simulink model "digitalControlSim"  (R2020a)
settings: Solver=VariableStepAuto  StartTime=0.0  StopTime=120  RelTol=1e-3
values from neighbouring files (symbols this model uses):
  Kp = 14.029    [digitalControlSyntesis.m]
  T = 1    [backwardDiscretization.m]    (also in backwardDiscretizationMultipleT.m = Tvec(k); digitalControlSyntesis.m = 0.1; discretizacion.m = Tvec(k); tustinDiscretization.m)
  Td = 12.5    [digitalControlSyntesis.m]
  Ti = 13.5593    [digitalControlSyntesis.m]
undefined symbols (not defined in the file or in its folder): den_back, den_tust, num_back, num_tust
libraries: simulink x1
settings Model: Creator=gbecerra  LastModifiedBy=gbecerra

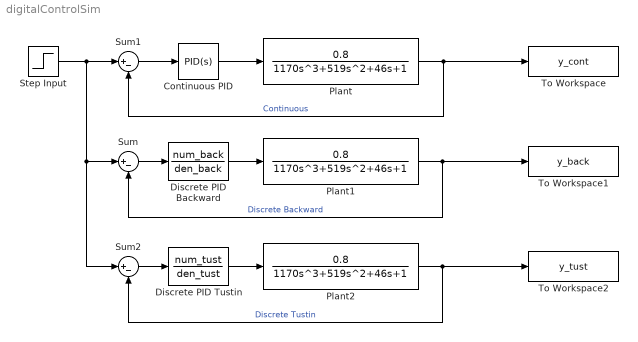
== system digitalControlSim ==
  Continuous PID : simulink/Continuous/PID Controller  Controller=PID  Form=Ideal  TimeDomain=Continuous-time  UseExternalTs=off  SampleTime=-1  IntegratorMethod=Forward Euler  FilterMethod=Forward Euler  ControllerParametersSource=internal  P=Kp  I=1/Ti  D=Td  UseFilter=on  N=100  TunerSelectOption=Transfer Function Based (PID Tuner App)  InitialConditionSource=internal  InitialConditionForIntegrator=0  InitialConditionForFilter=0  DifferentiatorICPrevScaledInput=0  ExternalReset=none  TrackingMode=off  Kt=1  LimitOutput=off  UpperSaturationLimit=inf  LowerSaturationLimit=-inf  LinearizeAsGain=on  AntiWindupMode=none  Kb=1  POutMin=[]  POutMax=[]  IOutMin=[]  IOutMax=[]  DOutMin=[]  DOutMax=[]  NOutMin=[]  NOutMax=[]  SumOutMin=[]  SumOutMax=[]  SaturationOutMin=[]  SaturationOutMax=[]  PParamMin=[]  PParamMax=[]  IParamMin=[]  IParamMax=[]  DParamMin=[]  DParamMax=[]  NParamMin=[]  NParamMax=[]  KbParamMin=[]  KbParamMax=[]  KtParamMin=[]  KtParamMax=[]  KbOutMin=[]  KbOutMax=[]  KtOutMin=[]  KtOutMax=[]  IntegratorOutMin=[]  IntegratorOutMax=[]  FilterOutMin=[]  FilterOutMax=[]  SumI1OutMin=[]  SumI1OutMax=[]  SumI2OutMin=[]  SumI2OutMax=[]  SumI3OutMin=[]  SumI3OutMax=[]  SumI4OutMin=[]  SumI4OutMax=[]  SumDOutMin=[]  SumDOutMax=[]  DifferentiatorOutMin=[]  DifferentiatorOutMax=[]  FilterDiffOutCoefMin=[]  FilterDiffOutCoefMax=[]  ReciprocalOutMin=[]  ReciprocalOutMax=[]  SumDenOutMin=[]  SumDenOutMax=[]  SumNumOutMin=[]  SumNumOutMax=[]  DivideOutMin=[]  DivideOutMax=[]  UdiffTsProdOutMin=[]  UdiffTsProdOutMax=[]  NTsProdOutMin=[]  NTsProdOutMax=[]  UintegralTsProdOutMin=[]  UintegralTsProdOutMax=[]  UngainTsProdOutMin=[]  UngainTsProdOutMax=[]  IntegratorContinuousStateAttributes=''  IntegratorStateMustResolveToSignalObject=off  IntegratorRTWStateStorageClass=Auto  FilterContinuousStateAttributes=''  FilterStateMustResolveToSignalObject=off  FilterRTWStateStorageClass=Auto  ParallelPVariant=Passthrough  IdealPVariant=InternalParameters  IVariant=InternalParameters  DVariant=InternalParameters  IntegratorVariant=Continuous  SatVariant=Disabled  AWVariant=Passthrough  PCopyVariant=Disabled  TRVariant=Disabled  FdbkBlocksVariant=Forward  IdealPFdbkVariant=Disabled  SatFdbkVariant=Disabled  DerivativeFilterVariant=ContFilter  NVariant=InternalParameters  NCopyVariant=Disabled  FilterICVariant=InternalICsFilter  IntegratorICVariant=InternalICs  ExternalResetVariant=Disabled  TRSumVariant=Passthrough  SumFdbkVariant=Disabled  SumVariant=Sum_PID  TsampFilterVariant=InternalTs  TsampNgainVariant=Passthrough  TsampIntegralVariant=Passthrough
  Discrete PID Backward : DiscreteTransferFcn  Numerator=num_back  Denominator=den_back  SampleTime=T
  Discrete PID Tustin : DiscreteTransferFcn  Numerator=num_tust  Denominator=den_tust  SampleTime=T
  Plant : TransferFcn  Numerator=0.8  Denominator=[1170 519 46 1]
  Plant1 : TransferFcn  Numerator=0.8  Denominator=[1170 519 46 1]
  Plant2 : TransferFcn  Numerator=0.8  Denominator=[1170 519 46 1]
  Step Input : Step  Time=0  SampleTime=0
  Sum : Sum  Inputs=|+-
  Sum1 : Sum  Inputs=|+-
  Sum2 : Sum  Inputs=|+-
  To Workspace : ToWorkspace  VariableName=y_cont  SaveFormat=Timeseries  SampleTime=-1
  To Workspace1 : ToWorkspace  VariableName=y_back  SaveFormat=Timeseries  SampleTime=-1
  To Workspace2 : ToWorkspace  VariableName=y_tust  SaveFormat=Timeseries  SampleTime=-1
  wires:
  Discrete PID Backward/1 -> Plant1/1
  Sum/1 -> Discrete PID Backward/1
  Step Input/1 -> Sum2/1, Sum/1, Sum1/1
  Plant1/1 -> To Workspace1/1, Sum/2  "Discrete Backward"
  Plant/1 -> To Workspace/1, Sum1/2  "Continuous"
  Sum1/1 -> Continuous PID/1
  Continuous PID/1 -> Plant/1
  Sum2/1 -> Discrete PID Tustin/1
  Discrete PID Tustin/1 -> Plant2/1
  Plant2/1 -> Sum2/2, To Workspace2/1  "Discrete Tustin"
